simulink model "problem2_sim"  (R2019a)
settings: Solver=FixedStepAuto  StartTime=0.0  StopTime=10.0  FixedStep=.01  RelTol=1e-3
values from neighbouring files (symbols this model uses):
  x_init = [x1_init(i), x2_init(i)]'    [problem_2.m]    (also in problem_3.m = [ 0.3, 0])
settings Model: Creator=glitch  LastModifiedBy=glitch

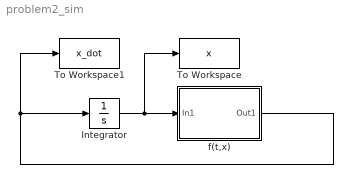
== system problem2_sim ==
  Integrator : Integrator  InitialCondition=x_init
  To Workspace : ToWorkspace  VariableName=x  SaveFormat=Structure With Time  SampleTime=-1
  To Workspace1 : ToWorkspace  VariableName=x_dot  SaveFormat=Structure With Time  SampleTime=-1
  f(t,x) : Subsystem
  wires:
  Integrator/1 -> f(t,x)/1(In1), To Workspace/1
  f(t,x)/1(Out1) -> Integrator/1, To Workspace1/1

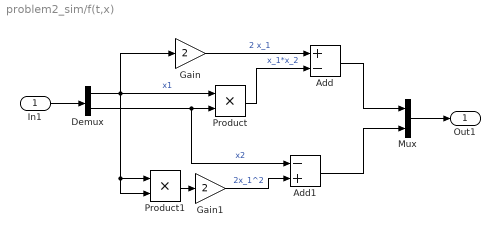
== system problem2_sim/f(t,x) ==
  In1 : Inport
  Add : Sum  Inputs=+-
  Add1 : Sum  Inputs=-+
  Demux : Demux  Outputs=2
  Gain : Gain  Gain=2
  Gain1 : Gain  Gain=2
  Mux : Mux  Inputs=2
  Product : Product
  Product1 : Product
  Out1 : Outport
  wires:
  Product1/1 -> Gain1/1
  Gain1/1 -> Add1/2  "2x_1^2"
  Add/1 -> Mux/1
  Mux/1 -> Out1/1
  Product/1 -> Add/2  "x_1*x_2"
  Gain/1 -> Add/1  "2 x_1"
  In1/1 -> Demux/1
  Demux/2 -> Add1/1, Product/2  "x2"
  Add1/1 -> Mux/2
  Demux/1 -> Product/1, Gain/1, Product1/2, Product1/1  "x1"
